simulink model "quarter_car"  (Simulink 7.0)
settings: Solver=ode4  StartTime=0.0  StopTime=5  FixedStep=0.001  RelTol=1e-3
settings Model: Creator=ibesseli  LastModifiedBy=ibesseli
settings DataIOCC: SignalLoggingName=sigsOut
settings DebuggingCC: SaveWithParameterizedLinksMsg=none  SignalResolutionControl=TryResolveAllWithWarning  SolverPrmCheckMsg=none  MultiTaskDSMMsg=warning  MultiTaskCondExecSysMsg=none  StrictBusMsg=None
settings HardwareCC: TargetUnknown=on
settings RTWCC: IncludeERTFirstTime=on
settings STFCustomTargetCC: GenFloatMathFcnCalls=ANSI_C  ModelReferenceCompliant=off  SystemTargetFile=grt.tlc

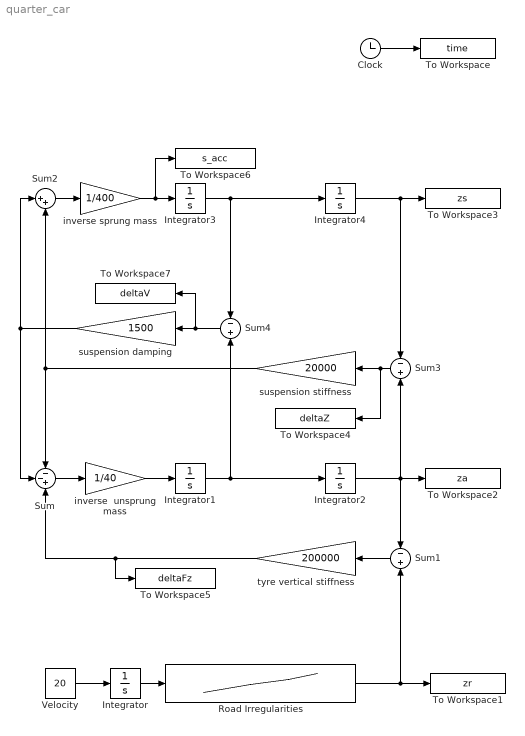
== system quarter_car ==
  Clock : Clock
      settings: Decimation=10
  Integrator{,1..4} (5 alike) : Integrator
  Road Irregularities : Lookup  InputValues=[0 10 10.01 50]  Table=[0 0 0.1 0.1]  OutDataType=sfix(16)  OutScaling=2^0  SaturateOnIntegerOverflow=on
  Sum : Sum  Inputs=--+  OutDataType=sfix(16)  OutScaling=2^0  SaturateOnIntegerOverflow=on
  Sum1 : Sum  Orientation=left  Inputs=-|+  OutDataType=sfix(16)  OutScaling=2^0  SaturateOnIntegerOverflow=on
  Sum2 : Sum  Inputs=|++  OutDataType=sfix(16)  OutScaling=2^0  SaturateOnIntegerOverflow=on
  Sum3 : Sum  Orientation=left  Inputs=-|+  OutDataType=sfix(16)  OutScaling=2^0  SaturateOnIntegerOverflow=on
  Sum4 : Sum  Orientation=left  Inputs=-|+  OutDataType=sfix(16)  OutScaling=2^0  SaturateOnIntegerOverflow=on
  To Workspace : ToWorkspace  VariableName=time  SampleTime=0.001  SaveFormat=Array
  To Workspace1 : ToWorkspace  VariableName=zr  SampleTime=-1  SaveFormat=Array
  To Workspace2 : ToWorkspace  VariableName=za  SampleTime=-1  SaveFormat=Array
  To Workspace3 : ToWorkspace  VariableName=zs  SampleTime=-1  SaveFormat=Array
  To Workspace4 : ToWorkspace  VariableName=deltaZ  SampleTime=0.001  SaveFormat=Array
  To Workspace5 : ToWorkspace  VariableName=deltaFz  SampleTime=0.001  SaveFormat=Array
  To Workspace6 : ToWorkspace  VariableName=s_acc  SampleTime=0.001  SaveFormat=Array
  To Workspace7 : ToWorkspace  VariableName=deltaV  SampleTime=0.001  SaveFormat=Array
  Velocity : Constant  Value=20  OutDataType=sfix(16)  OutScaling=2^0
  inverse sprung mass : Gain  Gain=1/400  ParameterDataType=sfix(16)  ParameterScaling=2^0  OutDataType=sfix(16)  OutScaling=2^0  SaturateOnIntegerOverflow=on
  inverse  unsprung mass : Gain  Gain=1/40  ParameterDataType=sfix(16)  ParameterScaling=2^0  OutDataType=sfix(16)  OutScaling=2^0  SaturateOnIntegerOverflow=on
  suspension damping : Gain  Orientation=left  Gain=1500  ParameterDataType=sfix(16)  ParameterScaling=2^0  OutDataType=sfix(16)  OutScaling=2^0  SaturateOnIntegerOverflow=on
  suspension stiffness : Gain  Orientation=left  Gain=20000  ParameterDataType=sfix(16)  ParameterScaling=2^0  OutDataType=sfix(16)  OutScaling=2^0  SaturateOnIntegerOverflow=on
  tyre vertical stiffness : Gain  Orientation=left  Gain=200000  ParameterDataType=sfix(16)  ParameterScaling=2^0  OutDataType=sfix(16)  OutScaling=2^0  SaturateOnIntegerOverflow=on
  wires:
  Integrator/1 -> Road Irregularities/1
  Velocity/1 -> Integrator/1
  Clock/1 -> To Workspace/1
  Road Irregularities/1 -> To Workspace1/1, Sum1/2
  Integrator1/1 -> Integrator2/1, Sum4/2
  Integrator2/1 -> To Workspace2/1, Sum1/1, Sum3/2
  Integrator3/1 -> Sum4/1, Integrator4/1
  Integrator4/1 -> To Workspace3/1, Sum3/1
  inverse sprung mass/1 -> Integrator3/1, To Workspace6/1
  inverse  unsprung mass/1 -> Integrator1/1
  Sum/1 -> inverse  unsprung mass/1
  Sum1/1 -> tyre vertical stiffness/1
  tyre vertical stiffness/1 -> Sum/3, To Workspace5/1
  Sum2/1 -> inverse sprung mass/1
  Sum3/1 -> suspension stiffness/1, To Workspace4/1
  suspension stiffness/1 -> Sum/1, Sum2/2
  Sum4/1 -> suspension damping/1, To Workspace7/1
  suspension damping/1 -> Sum/2, Sum2/1
